simulink model "CUAS_chart_modified"  (R2019b)
settings: Solver=VariableStepAuto  StartTime=0.0  StopTime=50  RelTol=1e-3
model workspace (MAT data in the model file):
  auth = 1
values from neighbouring files (symbols this model uses):
  Auth_DB_Check = 1.0    [test.sldd]
  ID_check = 0.0    [test.sldd]
  ID_DB_check = 0.0    [test.sldd]
  ID_validity_check = 0.0    [test.sldd]
  In_detection_range = 1.0    [test.sldd]
  P1 = 1.0    [test.sldd]
  P2 = 1.0    [test.sldd]
  P3 = 1.0    [test.sldd]
  P4 = 1.0    [test.sldd]
  P5 = 1.0    [test.sldd]
  P6 = 1.0    [test.sldd]
  P7 = 1.0    [test.sldd]
  P8 = 1.0    [test.sldd]
  T_Area = 1.0    [test.sldd]
  T_AUTH_CUAS = 1.0    [test.sldd]
  T_AUTH_DB = 1.0    [test.sldd]
  T_AUTH_USS = 1.0    [test.sldd]
  T_ID_DB = 1.0    [test.sldd]
  T_ID_Read = 1.0    [test.sldd]
  T_ID_valid = 1.0    [test.sldd]
  T_resp_delay = 1.0    [test.sldd]
  T_time = 1.0    [test.sldd]
  T_timeout = 5.0    [test.sldd]
  T_timeout_inerdict = 5.0    [test.sldd]
  T_verifyID = 1.0    [test.sldd]
  Time_check = 0.0    [test.sldd]
  verify_ID = 0.0    [test.sldd]
  Zone_check = 0.0    [test.sldd]
libraries: simulink x1
settings Model: DataDictionary=test.sldd  EnablePacing=on  Creator=ruba.alkadi  LastModifiedBy=ruba.alkadi
settings DataIOCC: ExternalInput=c

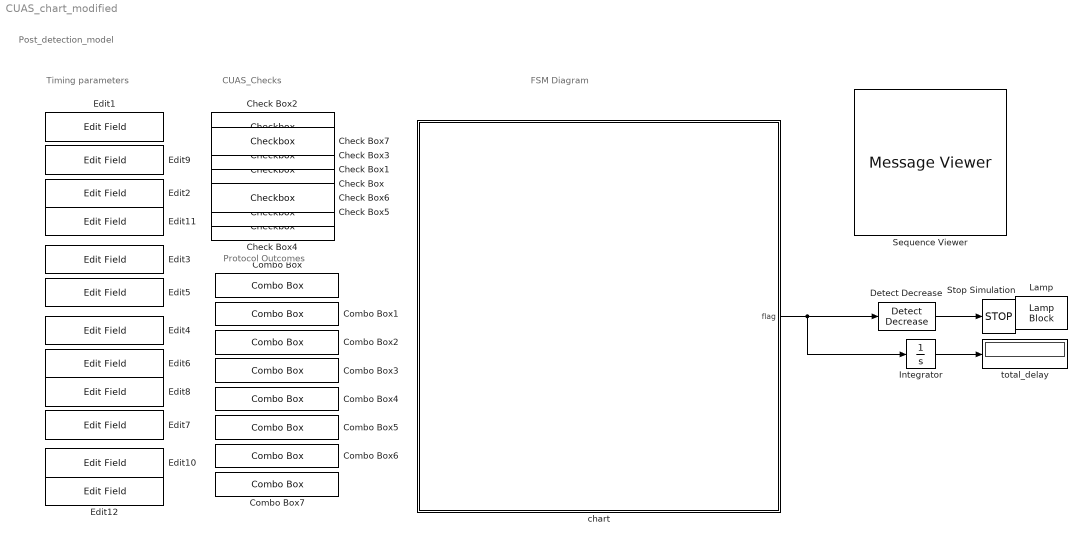
== system CUAS_chart_modified ==
  note: CUAS_Checks
  note: FSM Diagram
  note: Timing parameters
  note: Protocol Outcomes
  note: Post_detection_model
  Check Box : Checkbox  LabelPosition=Hide  ShowInitialText=on  Label=Check_AUTH_DB
  Check Box1 : Checkbox  LabelPosition=Hide  ShowInitialText=on  Label=Check_ID_DB
  Check Box2 : Checkbox  LabelPosition=Hide  ShowInitialText=on  Label=Check_ID
  Check Box3 : Checkbox  LabelPosition=Hide  ShowInitialText=on  Label=ID_validity_check
  Check Box4 : Checkbox  LabelPosition=Hide  ShowInitialText=on  Label=In_detection_range
  Check Box5 : Checkbox  LabelPosition=Hide  ShowInitialText=on  Label=Check_AUTH_Time
  Check Box6 : Checkbox  LabelPosition=Hide  ShowInitialText=on  Label=Check_AUTH_Area
  Check Box7 : Checkbox  LabelPosition=Hide  ShowInitialText=on  Label=Verify_ID
  Combo Box : ComboBox  LabelPosition=Hide  SelectedLabel=P1_1
      settings: Values={{'P1_1', 'P1_2', 'P1_3', 'P1_4', 'P1_5'}, [1 2 3 4 5]}
  Combo Box1 : ComboBox  LabelPosition=Hide  SelectedLabel=P2_1
      settings: Values={{'P2_1', 'P2_2', 'P2_3'}, [1 2 3]}
  Combo Box2 : ComboBox  LabelPosition=Hide  SelectedLabel=P3_1
      settings: Values={{'P3_1', 'P3_2'}, [1 2]}
  Combo Box3 : ComboBox  LabelPosition=Hide  SelectedLabel=P4_1
      settings: Values={{'P4_1', 'P4_2'}, [1 2]}
  Combo Box4 : ComboBox  LabelPosition=Hide  SelectedLabel=P5_1
      settings: Values={{'P5_1', 'P5_2'}, [1 2]}
  Combo Box5 : ComboBox  LabelPosition=Hide  SelectedLabel=P6_1
      settings: Values={{'P6_1', 'P6_2', 'P6_3'}, [1 2 3]}
  Combo Box6 : ComboBox  LabelPosition=Hide  SelectedLabel=P7_1
      settings: Values={{'P7_1', 'P7_2', 'P7_3'}, [1 2 3]}
  Combo Box7 : ComboBox  LabelPosition=Hide  SelectedLabel=P8_1
      settings: Values={{'P8_1', 'P8_2', 'P8_3'}, [1 2 3]}
  Detect Decrease : simulink/Logic and Bit Operations/Detect Decrease  vinit=0  OutDataTypeStr=boolean
  Edit{1..12} (12 alike) : EditField  ShowInitialText=on  Alignment=Center
  Integrator : Integrator
  Lamp : LampBlock  LabelPosition=Hide
  Sequence Viewer : MessageViewer
  Stop Simulation : Stop
  chart : Stateflow chart  BlockKeywords=__PRM__SERIALIZED__DATA__:Stateflow Chart,Stateflow Diagram  TreatAsAtomicUnit=on
  total_delay : Display
  wires:
  Detect Decrease/1 -> Stop Simulation/1
  chart/1(flag) -> Integrator/1, Detect Decrease/1
  Integrator/1 -> total_delay/1

== stateflow chart CUAS_chart_modified/chart ==
  state Tolerate_ID_failure
    Tolerate_ID=1
  state Tolerate_AUTH_Failure
    Tolerate_Auth=1
  state mission_within_time
    flag=0;
  state Authorized_mission
  state drone_detected
    flag=1;
  state ID_received
  state Authentic_ID
  state mission_within_zone
  state mission_out_of_range
  state Valid_ID
  state Known_ID
  state Survaillance
    flag=0
  state No_ID_received
  state No_ID_received1_potential_Opr
    P1
    T_P1_C1= T_AUTH_CUAS +2* T_resp_delay + 2*T_AUTH_USS + T_timeout ;
    T_P1_C2= T_AUTH_CUAS +3* T_resp_delay + T_AUTH_USS ;
    T_P1_C3_4= T_AUTH_CUAS +2* T_AUTH_USS + T_AUTH_CUAS +3* T_resp_delay ;
    T_P1_C5=3* T_AUTH_CUAS +2* T_AUTH_USS + T_AUTH_CUAS + T_AUTH_CUAS +5* T_resp_delay ;
  state Area_violation
    P7
    T_P7_C1= T_AUTH_CUAS + T_resp_delay +2* T_AUTH_USS + T_timeout + T_timeout_inerdict ;
    T_P7_C2_3= T_AUTH_CUAS +3* T_resp_delay +3* T_AUTH_USS + T_timeout_inerdict ;
    T_P7_C4=2* T_AUTH_USS +3* T_resp_delay +2* T_AUTH_CUAS ;
  state Time_violation
    P8
    T_P8_C1= T_AUTH_CUAS + T_resp_delay +2* T_AUTH_USS + T_timeout + T_timeout_inerdict ;
    T_P8_C2_3= T_AUTH_CUAS +3* T_resp_delay +3* T_AUTH_USS + T_timeout_inerdict ;
    T_P8_C3=2* T_AUTH_USS +3* T_resp_delay +2* T_AUTH_CUAS ;
  state No_ID_received_No_potential_operator
    flag=1;
  state Fake_ID
  state ID_not_in_IDDB
  state ID_in_AUTHDB
    P3
    T_P3_C1= T_AUTH_CUAS + T_resp_delay ;
    T_P3_C2= T_AUTH_CUAS + T_resp_delay + T_AUTH_USS  + T_timeout_inerdict ;
  state Expired_ID_authorized
    P5
  state Expired_ID
  state UnAuthorized
    P6
    T_P6_C1=2* T_AUTH_CUAS + T_resp_delay ;
    T_P6_C2= T_AUTH_CUAS + T_resp_delay + T_AUTH_USS  + T_timeout_inerdict ;
    T_P6_C3= T_resp_delay +2* T_AUTH_CUAS ;
  state Unknown_ID
    P2
    T_P2_C1= T_AUTH_CUAS + T_resp_delay ;
    T_P2_C2= T_AUTH_CUAS + T_resp_delay + T_AUTH_USS  + T_timeout_inerdict ;
    T_P2_C3= T_AUTH_CUAS + T_resp_delay + T_AUTH_USS ;
  state Expired_ID_and_unauthorized
    P4
  state Immediate_Interdiction
    flag=0;
  state Delayed_interdiction
    flag=0;
  mission_out_of_range -> Survaillance : [In_detection_range==0]
  mission_within_time -> drone_detected [order 4] : [In_detection_range==1]
  mission_within_time -> Tolerate_ID_failure [order 3] : [In_detection_range==1&&Tolerate_ID==1]
  Tolerate_ID_failure -> Authorized_mission [order 2] : [Auth_DB_Check==1]
  No_ID_received1_potential_Opr -> Tolerate_ID_failure [order 4] : [P1==3||P1==4]
  Tolerate_AUTH_Failure -> mission_within_zone [order 2] : [Zone_check==1]
  Tolerate_AUTH_Failure -> Area_violation [order 1] : [Zone_check==0]
  mission_within_time -> Tolerate_AUTH_Failure [order 2] : [In_detection_range==1&&Tolerate_Auth==1]
  Area_violation -> Tolerate_AUTH_Failure [order 2] : after(T_P7_C2_3,sec)[P7==2||P7==3]
  Expired_ID_authorized -> Tolerate_ID_failure [order 2] : after(T_resp_delay,sec)[P5==2]
  Unknown_ID -> Tolerate_AUTH_Failure [order 1] : after(T_P2_C3,sec)[P2==3]
  ID_in_AUTHDB -> Tolerate_ID_failure [order 2] : after(T_P3_C2,sec)[P3==2]
  Tolerate_ID_failure -> UnAuthorized [order 1] : [Auth_DB_Check==0]
  Expired_ID_and_unauthorized -> Tolerate_AUTH_Failure [order 1] : after(T_resp_delay,sec)[P4==2]
  UnAuthorized -> Tolerate_AUTH_Failure [order 3] : after(T_P6_C3,sec)[P6==3]
  (default) -> Survaillance
  mission_within_zone -> mission_within_time [order 1] : after(T_time,sec)[Time_check==1]
  mission_within_time -> mission_out_of_range [order 1] : [In_detection_range==0]
  drone_detected -> ID_received [order 1] : after(T_ID_Read,sec)[ID_check==1]
  Survaillance -> drone_detected : [In_detection_range==1]
  ID_received -> Authentic_ID [order 1] : after(T_verifyID,sec)[verify_ID==1]
  Authorized_mission -> mission_within_zone [order 1] : after(T_Area,sec)[Zone_check==1]
  Valid_ID -> Authorized_mission [order 1] : after(T_AUTH_DB,sec)[Auth_DB_Check==1]
  Authentic_ID -> Known_ID [order 1] : after(T_ID_DB,sec)[ID_DB_check==1]
  Known_ID -> Valid_ID [order 1] : after(T_ID_valid,sec)[ID_validity_check==1]
  Delayed_interdiction -> Survaillance
  UnAuthorized -> Authorized_mission [order 1] : after(T_P6_C1,sec)[P6==1]
  ID_in_AUTHDB -> Known_ID [order 1] : after(T_P3_C1,sec)[P3==1]
  Time_violation -> mission_within_time [order 3] : after(T_P8_C2_3,sec)[P8==2]
  drone_detected -> No_ID_received [order 2] : after(T_ID_Read,sec)[ID_check==0]
  Area_violation -> mission_within_zone [order 1] : after(T_P7_C1,sec)[P7==1]
  Known_ID -> Expired_ID [order 2] : after(T_ID_valid,sec)[ID_validity_check==0]
  Expired_ID_authorized -> Valid_ID [order 1] : after(T_resp_delay,sec)[P5==1]
  Valid_ID -> UnAuthorized [order 2] : after(T_AUTH_DB,sec)[Auth_DB_Check==0]
  No_ID_received1_potential_Opr -> ID_received [order 3] : after(T_P1_C5,sec)[P1==5]
  ID_received -> Fake_ID [order 2] : after(T_verifyID,sec)[verify_ID==0]
  Authentic_ID -> ID_not_in_IDDB [order 2] : after(T_ID_DB,sec)[ID_DB_check==0]
  Time_violation -> mission_out_of_range [order 1] : after(T_P8_C3,sec)[P8==3]
  Authorized_mission -> Area_violation [order 2] : after(T_Area,sec)[Zone_check==0]
  mission_within_zone -> Time_violation [order 2] : after(T_time,sec)[Time_check==1]
  Immediate_Interdiction -> Survaillance
  No_ID_received -> No_ID_received1_potential_Opr [order 1] : after(T_AUTH_DB,sec)[Auth_DB_Check==1]
  No_ID_received1_potential_Opr -> Immediate_Interdiction [order 1] : after(max(T_P1_C1,T_P1_C2),sec)[P1==1||P1==2]
  No_ID_received -> No_ID_received_No_potential_operator [order 2] : after(T_AUTH_DB,sec)[Auth_DB_Check==0]
  No_ID_received1_potential_Opr -> Delayed_interdiction [order 2] : after(T_P1_C3_4,sec)[P1==3||P1==4]
  ID_not_in_IDDB -> ID_in_AUTHDB [order 1] : after(T_AUTH_DB,sec)[Auth_DB_Check==1]
  Expired_ID -> Expired_ID_authorized [order 2] : after(T_AUTH_DB,sec)[Auth_DB_Check==1]
  Expired_ID -> Expired_ID_and_unauthorized [order 1] : after(T_AUTH_DB,sec)[Auth_DB_Check==0]
  No_ID_received_No_potential_operator -> Immediate_Interdiction
  Fake_ID -> Immediate_Interdiction
  ID_not_in_IDDB -> Unknown_ID [order 2] : after(T_AUTH_DB,sec)[Auth_DB_Check==0]
  Area_violation -> Delayed_interdiction [order 3] : after(T_P7_C2_3,sec)[P7==4]
  Time_violation -> Delayed_interdiction [order 2] : after(T_P8_C1,sec)[P8==1]
  UnAuthorized -> Delayed_interdiction [order 2] : after(T_P6_C2,sec)[P6==2]
  Unknown_ID -> Delayed_interdiction [order 3] : after(T_P2_C2,sec)[P2==2]
  Unknown_ID -> Immediate_Interdiction [order 2] : after(T_P2_C1,sec)[P2==1]
  Expired_ID_and_unauthorized -> Delayed_interdiction [order 2] : after(T_timeout_inerdict,sec)[P4==1]
  data: Tolerate_Auth local =0; Tolerate_ID local =0; P1 parameter; Auth_DB_Check parameter; P8 parameter; P7 parameter; P2 parameter; P3 parameter; P4 parameter; P5 parameter; P6 parameter; verify_ID parameter; Zone_check parameter; Time_check parameter; In_detection_range parameter; ID_validity_check parameter; ID_check parameter; ID_DB_check parameter; flag output =0; T_ID_Read parameter; T_AUTH_USS parameter; T_AUTH_DB parameter; T_P1_C2 local; T_P1_C1 local; T_P1_C5 local; T_P1_C3_4 local; T_timeout parameter; T_resp_delay parameter; T_AUTH_CUAS parameter; T_verifyID parameter; T_ID_DB parameter; T_P2_C2 local; T_P2_C1 local; T_P2_C3 local; T_timeout_inerdict parameter; T_ID_valid parameter; T_P3_C1 local; T_P3_C2 local; T_P6_C1 local; T_P6_C2 local; T_P6_C3 local; T_P8_C2_3 local; T_P7_C4 local; T_time parameter; T_Area parameter; T_P7_C1 local; T_P7_C2_3 local; T_P8_C1 local; T_P8_C3 local
